simulink model "xpcUEIFrame"  (Simulink 6.0)
settings: Solver=FixedStepDiscrete  SolverMode=SingleTasking  StartTime=0.0  StopTime=inf  RelTol=1e-3
undefined symbols (not defined in the file or in its folder): MF, PD2
libraries: dspsigattribs x2, xpclib x2
settings Model: Creator=gweast  LastModifiedBy=ekbas  ExtModeArmWhenConnect=off  BufferReuse=off  ProdHWDeviceType=Specified
settings DataIOCC: SignalLoggingName=sigsOut
settings OptimizationCC: BooleanDataType=off  InlineInvariantSignals=off  OptimizeBlockIOStorage=off  BufferReuse=off  EnforceIntegerDowncast=off  FoldNonRolledExpr=off  LocalBlockOutputs=off  MultiInstanced=off
settings FormatCC: IgnoreBidirectionalLines=off
settings HardwareCC: ProdHWDeviceType=Specified
settings RTWCC: SystemTargetFile=xpctarget.tlc  TemplateMakefile=xpc_default_tmf  ProcessScript=xpctarget_make_rtw_hook
settings CodeAppCC: SimulinkBlockComments=off
settings xpcTargetCC: TargetFcnLib=iso_c_tmw.mat

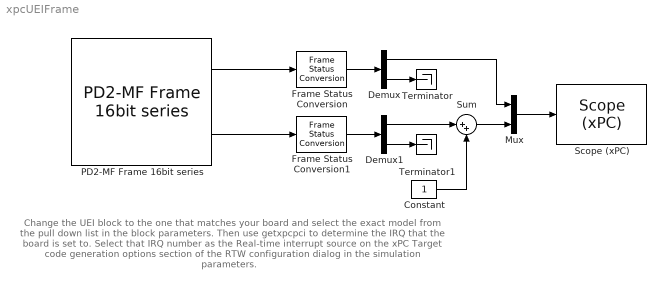
== system xpcUEIFrame ==
  note: Change the UEI block to the one that matches your board and
      | select the exact model from the pull down list in the block
      | parameters.  Then use getxpcpci to determine the IRQ that
      | the board is set to.  Select that IRQ number as the Real-time
      | interrupt source on the xPC Target code generation options
      | section of the RTW configuration dialog in the simulation
      | parameters.
  Constant : Constant
  Demux : Demux  Outputs=[1 -1]
  Demux1 : Demux  Outputs=[1 -1]
  Frame Status Conversion : dspsigattribs/Frame Status Conversion  growRefPort=off  outframe=Sample-based
  Frame Status Conversion1 : dspsigattribs/Frame Status Conversion  growRefPort=off  outframe=Sample-based
  Mux : Mux  Inputs=2
  "PD2-MF Frame 16bit series " : xpclib/A//D Frame/UEI/PD2-MF Frame 16bit series   boardtypein=PD2-MF-16-333/16H  channel=[1 2]  gain=[1]  mux=[0]  range=+- 10 Volts  sediff=Single Ended  framesize=32  outfmt=Frame (Signal Processing blockset needed)  clsource=Internal  scantime=-1  frametime=0.001  sampletime=off  slave=off  freq=-1  burst=32  pcislot=-1
  "Scope (xPC) " : xpclib/Misc./Scope (xPC)   scopeno=1  scopetype=Target  autostart=on  viewmode=Graphical redraw  formatstr='%15.6f'  grid=on  ylimits=[0,0]  nosamples=100  noprepostsamples=0  interleave=1  triggermode=FreeRun  triggersignal=1  triggerlevel=0.0  triggerslope=Either  triggerscope=1  triggersample=0  filename=data.dat  mode=Lazy  writesize=512  autorestart=off
  Sum : Sum  Inputs=|++  SaturateOnIntegerOverflow=on
  Terminator : Terminator
  Terminator1 : Terminator
  wires:
  "PD2-MF Frame 16bit series "/1 -> Frame Status Conversion/1
  Frame Status Conversion/1 -> Demux/1
  Demux/2 -> Terminator/1
  "PD2-MF Frame 16bit series "/2 -> Frame Status Conversion1/1
  Frame Status Conversion1/1 -> Demux1/1
  Demux1/2 -> Terminator1/1
  Demux/1 -> Mux/1
  Mux/1 -> "Scope (xPC) "/1
  Demux1/1 -> Sum/1
  Sum/1 -> Mux/2
  Constant/1 -> Sum/2
